simulink model "xiti4_8_10T3"  (Simulink 5.0)
settings: Solver=ode45  StartTime=0.0  StopTime=200  FixedStep=0.01  RelTol=1e-3
libraries: simulink_extras x2
CloseFcn:
  | rtwprivate ssgensfun ModelCloseRequest PID_PI
settings Model: LastModifiedBy=ThinkPad

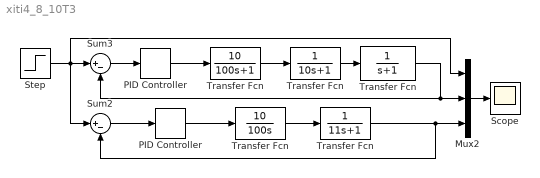
== system xiti4_8_10T3 ==
  " Transfer Fcn" : TransferFcn  Numerator=[10]  Denominator=[100 0]
  " Transfer Fcn " : TransferFcn  Denominator=[10 1]
  " Transfer Fcn  " : TransferFcn  Numerator=[10]  Denominator=[100 1]
  Mux2 : Mux  Inputs=3
  PID Controller : simulink_extras/Additional Linear/PID Controller  P=1  I=0  D=0
  "PID Controller " : simulink_extras/Additional Linear/PID Controller  P=1  I=0  D=0
  Scope : Scope
      settings: TimeRange=300  YMin=0  YMax=1.4  SaveName=xiti4_83  DataFormat=Array  MaxDataPoints=500000
  "Step " : Step  Time=0  SampleTime=0
  Sum2 : Sum  Inputs=|+-  SaturateOnIntegerOverflow=on
  Sum3 : Sum  Inputs=|+-  SaturateOnIntegerOverflow=on
  Transfer Fcn : TransferFcn  Denominator=[11 1]
  "Transfer Fcn " : TransferFcn  Denominator=[1 1]
  wires:
  "Step "/1 -> Sum2/1, Sum3/1, Mux2/1
  Sum3/1 -> "PID Controller "/1
  "PID Controller "/1 -> " Transfer Fcn  "/1
  " Transfer Fcn "/1 -> "Transfer Fcn "/1
  Sum2/1 -> PID Controller/1
  PID Controller/1 -> " Transfer Fcn"/1
  Mux2/1 -> Scope/1
  "Transfer Fcn "/1 -> Sum3/2, Mux2/2
  " Transfer Fcn  "/1 -> " Transfer Fcn "/1
  Transfer Fcn/1 -> Sum2/2, Mux2/3
  " Transfer Fcn"/1 -> Transfer Fcn/1
